simulink model "LQRSimulinkLongWind"  (R2025b)
settings: Solver=VariableStepAuto  StartTime=0.0  StopTime=100  RelTol=1e-3
undefined symbols (not defined in the file): A_long, B_long, K_long
settings Model: Creator=leonardoleggeri  LastModifiedBy=leonardoleggeri

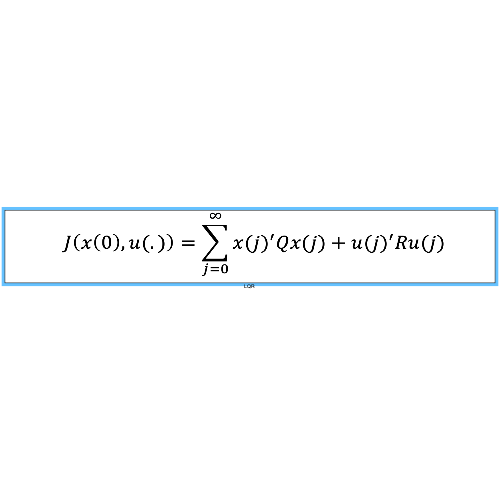
[thumbnail: Simulink's stored preview of the top-level diagram]
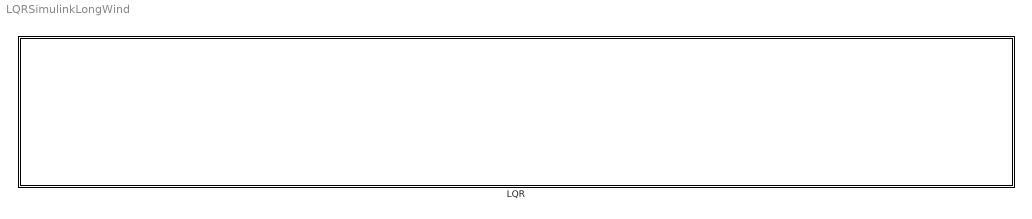
== system LQRSimulinkLongWind ==
  LQR : Subsystem
      mask Display: image('LQR.png');

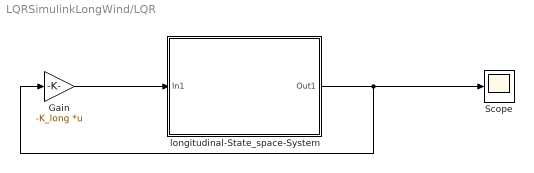
== system LQRSimulinkLongWind/LQR ==
  Gain : Gain  Gain=-K_long  Multiplication=Matrix(K*u)
  Scope : Scope
      settings: ActiveDisplayYMinimum=-0.18974322374260028  ActiveDisplayYMaximum=0.17739989371994563
  longitudinal-State_space-System : Subsystem
      mask Display: image('F16_SCANG_InFlight.jpg');
  wires:
  Gain/1 -> longitudinal-State_space-System/1(In1)
  longitudinal-State_space-System/1(Out1) -> Scope/1, Gain/1

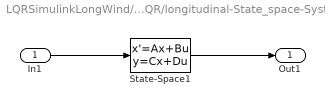
== system LQRSimulinkLongWind/LQR/longitudinal-State_space-System ==
  In1 : Inport
  State-Space1 : StateSpace  A=A_long  B=B_long  C=eye(4)  D=zeros(4,5)  InitialCondition=[0.8; 0.6; 50; 15]
  Out1 : Outport
  wires:
  In1/1 -> State-Space1/1
  State-Space1/1 -> Out1/1
